simulink model "gm_Approximate_id_0af2ac3f3b928182f3ff557fc379a1d7491938e9"  (R2020a)
settings: Solver=VariableStepAuto  StartTime=0.0  StopTime=10.0  RelTol=1e-3
model workspace (MAT data in the model file):
  InputValues_20210824T100641914 = [-5; -4.9375; -4.875; -4.8125; -4.75; -4.6875; -4.625; -4.5625; -4.5; -4.4375; -4.375; -4.3125; -4.25; -4.1875; -4.125; -4.0625; -4; -3.9375; -3.875; -3.8125; -3.75; -3.6875; -3.625; -3.5625; -3.5; -3.4375; -3.375; -3.3125; -3.25; -3.1875; -3.125; -3.0625; -3; -2.9375; -2.875; -2.8125; -2.75; -2.6875; -2.625; -2.5625; -2.5; -2.4375; -2.375; -2.3125; -2.25; -2.1875; -2.125; -2.0625; -2; -1.9375; -1.875; -1.8125; -1.75; -1.6875; -1.625; -1.5625; -1.5; -1.4375; -1.375; -1.3125; -1.25; -1.1875; -1.125; -1.0625; -1; -0.9375; -0.875; -0.8125; -0.75; -0.6875; -0.625; -0.5625; -0.5; -0.4375; -0.375; -0.3125; -0.25; -0.1875; -0.125; -0.0625; 0; 0.0625; 0.125; 0.1875; 0.25; 0.3125; 0.375; 0.4375; 0.5; 0.5625; 0.625; 0.6875; 0.75; 0.8125; 0.875; 0.9375; 1; 1.0625; 1.125; 1.1875; 1.25; 1.3125; 1.375; 1.4375; 1.5; 1.5625; 1.625; 1.6875; 1.75; 1.8125; 1.875; 1.9375; 2; 2.0625; 2.125; 2.1875; 2.25; 2.3125; 2.375; 2.4375; 2.5; 2.5625; 2.625; 2.6875; 2.75; 2.8125; 2.875; 2.9375; 3; 3.0625; 3.125; 3.1875; 3.25; 3.3125; 3.375; 3.4375; 3.5; 3.5625; 3.625; 3.6875; 3.75; 3.8125; 3.875; 3.9375; 4; 4.0625; 4.125; 4.1875; 4.25; 4.3125; 4.375; 4.4375; 4.5; 4.5625; 4.625; 4.6875; 4.75; 4.8125; 4.875; 4.9375; 5]
settings Model: Creator=Mahsa  LastModifiedBy=Mahsa
settings OptimizationCC: BlockReduction=off  ConditionallyExecuteInputs=off
settings DebuggingCC: InheritedTsInSrcMsg=none

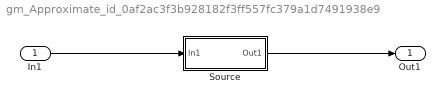
== system gm_Approximate_id_0af2ac3f3b928182f3ff557fc379a1d7491938e9 ==
  In1 : Inport  OutDataTypeStr=fixdt(1, 8, 4)  PortDimensions=1  SampleTime=0
  Source : Subsystem
  Out1 : Outport
  wires:
  In1/1 -> Source/1(In1)
  Source/1(Out1) -> Out1/1

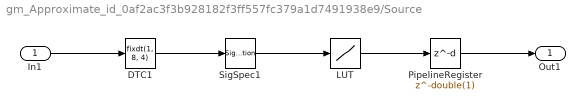
== system gm_Approximate_id_0af2ac3f3b928182f3ff557fc379a1d7491938e9/Source ==
  In1 : Inport  OutDataTypeStr=fixdt(1, 8, 4)  PortDimensions=1  SampleTime=0
  DTC1 : DataTypeConversion  OutDataTypeStr=fixdt(1, 8, 4)  RndMeth=Nearest  SampleTime=0
  LUT : Lookup_n-D  NumberOfTableDimensions=1  BreakpointsForDimension1="fi(\"numerictype\",numerictype(1,8,4),\"fimath\",fimath(\"RoundingMethod\", \"Floor\",\"OverflowAction\", \"Wrap\",\"ProductMode\",\"FullPrecision\",\"SumMode\",\"FullPrecision\"),\"Value\",\"[-5 -4.9375 -4.875 -4.8125 -4.75 -4.6875 -4.625 -4.5625 -4.5 -4.4375 -4.375 -4.3125 -4.25 -4.1875 -4.125 -4.0625 -4 -3.9375 -3.875 -3.8125 -3.75 -3.6875 -3.625 -3.5625 -3.5 -3.4375 -3.375 -3.3125 -3.25 -3.1875 -3.125 -3.0625 -3 -2.9375 -2.875 -2.8125 -2.75 -2.6875 -2.625 -2.5625 -2.5 -2.4375 -2.375 -2.3125 -2.25 -2.1875 -2.125 -2.0625 -2 -1.9375 -1.875 -1.8125 -1.75 -1.6875 -1.625 -1.5625 -1.5 -1.4375 -1.375 -1.3125 -1.25 -1.1875 -1.125 -1.0625 -1 -0.9375 -0.875 -0.8125 -0.75 -0.6875 -0.625 -0.5625 -0.5 -0.4375 -0.375 -0.3125 -0.25 -0.1875 -0.125 -0.0625 0 0.0625 0.125 0.1875 0.25 0.3125 0.375 0.4375 0.5 0.5625 0.625 0.6875 0.75 0.8125 0.875 0.9375 1 1.0625 1.125 1.1875 1.25 1.3125 1.375 1.4375 1.5 1.5625 1.625 1.6875 1.75 1.8125 1.875 1.9375 2 2.0625 2.125 2.1875 2.25 2.3125 2.375 2.4375 2.5 2.5625 2.625 2.6875 2.75 2.8125 2.875 2.9375 3 3.0625 3.125 3.1875 3.25 3.3125 3.375 3.4375 3.5 3.5625 3.625 3.6875 3.75 3.8125 3.875 3.9375 4 4.0625 4.125 4.1875 4.25 4.3125 4.375 4.4375 4.5 4.5625 4.625 4.6875 4.75 4.8125 4.875]\")"  Table="reshape(fi(\"numerictype\",numerictype(1,8,7),\"fimath\",fimath(\"RoundingMethod\", \"Floor\",\"OverflowAction\", \"Wrap\",\"ProductMode\",\"FullPrecision\",\"SumMode\",\"FullPrecision\"),\"Value\",\"[-1;-1;-1;-1;-1;-1;-1;-1;-1;-1;-1;-1;-1;-1;-1;-1;-1;-1;-1;-1;-1;-1;-1;-1;-1;-1;-1;-1;-1;-1;-1;-0.9921875;-0.9921875;-0.9921875;-0.9921875;-0.9921875;-0.9921875;-0.9921875;-0.9921875;-0.984375;-0.984375;-0.984375;-0.984375;-0.984375;-0.9765625;-0.9765625;-0.96875;-0.96875;-0.9609375;-0.9609375;-0.953125;-0.9453125;-0.9375;-0.9375;-0.921875;-0.9140625;-0.90625;-0.890625;-0.8828125;-0.8671875;-0.8515625;-0.828125;-0.8125;-0.7890625;-0.7578125;-0.734375;-0.703125;-0.671875;-0.6328125;-0.59375;-0.5546875;-0.5078125;-0.4609375;-0.4140625;-0.359375;-0.3046875;-0.2421875;-0.1875;-0.125;-0.0625;0;0.0625;0.125;0.1875;0.2421875;0.3046875;0.359375;0.4140625;0.4609375;0.5078125;0.5546875;0.59375;0.6328125;0.671875;0.703125;0.734375;0.7578125;0.7890625;0.8125;0.828125;0.8515625;0.8671875;0.8828125;0.890625;0.90625;0.9140625;0.921875;0.9375;0.9375;0.9453125;0.953125;0.9609375;0.9609375;0.96875;0.96875;0.9765625;0.9765625;0.984375;0.984375;0.984375;0.984375;0.984375;0.9921875;0.9921875;0.9921875;0.9921875;0.9921875;0.9921875;0.9921875;0.9921875;0.9921875;0.9921875;0.9921875;0.9921875;0.9921875;0.9921875;0.9921875;0.9921875;0.9921875;0.9921875;0.9921875;0.9921875;0.9921875;0.9921875;0.9921875;0.9921875;0.9921875;0.9921875;0.9921875;0.9921875;0.9921875;0.9921875;0.9921875;0.9921875;0.9921875;0.9921875;0.9921875;0.9921875;0.9921875]\"), [1  159])"  InterpMethod=Flat  ExtrapMethod=Clip  SampleTime=0  OutDataTypeStr=fixdt(1, 8, 7)  RndMeth=Simplest  InputSameDT=on
  PipelineRegister : Delay  DelayLength=double(1)  InitialCondition=0
  SigSpec1 : SignalSpecification  OutDataTypeStr=fixdt(1, 8, 4)  Dimensions=1
  Out1 : Outport
  wires:
  In1/1 -> DTC1/1
  DTC1/1 -> SigSpec1/1
  PipelineRegister/1 -> Out1/1
  SigSpec1/1 -> LUT/1
  LUT/1 -> PipelineRegister/1
